simulink model "EVModeling"  (R2024b)
settings: Solver=ode23tb  StartTime=0  StopTime=1800  RelTol=1e-3
model workspace (MAT data in the model file):
  Af = Simulink.Parameter
  Af.Value = 2.27
  Af.Complexity = 'real'
  Af.Dimensions = [1 1]
  Af.DataType = 'double'
  Bx = Simulink.Parameter
  Bx.Value = 10
  Bx.Complexity = 'real'
  Bx.Dimensions = [1 1]
  Bx.DataType = 'double'
  CI = 0.1
  Cd = Simulink.Parameter
  Cd.Value = 0.28
  Cd.Complexity = 'real'
  Cd.Dimensions = [1 1]
  Cd.DataType = 'double'
  Cl = Simulink.Parameter
  Cl.Value = 0.1
  Cl.Complexity = 'real'
  Cl.Dimensions = [1 1]
  Cl.DataType = 'double'
  Cpm = Simulink.Parameter
  Cpm.Value = 0.1
  Cpm.Complexity = 'real'
  Cpm.Dimensions = [1 1]
  Cpm.DataType = 'double'
  Cx = Simulink.Parameter
  Cx.Value = 1.65
  Cx.Complexity = 'real'
  Cx.Dimensions = [1 1]
  Cx.DataType = 'double'
  Dx = Simulink.Parameter
  Dx.Value = 1
  Dx.Complexity = 'real'
  Dx.Dimensions = [1 1]
  Dx.DataType = 'double'
  Ex = Simulink.Parameter
  Ex.Value = 0.01
  Ex.Complexity = 'real'
  Ex.Dimensions = [1 1]
  Ex.DataType = 'double'
  FZMAX = Simulink.Parameter
  FZMAX.Value = 6570
  FZMAX.Complexity = 'real'
  FZMAX.Dimensions = [1 1]
  FZMAX.DataType = 'double'
  FZMIN = Simulink.Parameter
  FZMIN.Value = 0
  FZMIN.Complexity = 'real'
  FZMIN.Dimensions = [1 1]
  FZMIN.DataType = 'double'
  Fc = Simulink.Parameter
  Fc.Value = 500
  Fc.Complexity = 'real'
  Fc.Dimensions = [1 1]
  Fc.DataType = 'double'
  FsbF = Simulink.Parameter
  FsbF.Value = [-700000 -7000 -700 0 700 7000 700000]
  FsbF.Complexity = 'real'
  FsbF.Dimensions = [1 7]
  FsbF.DataType = 'double'
  FsbR = Simulink.Parameter
  FsbR.Value = [-700000 -7000 -700 0 700 7000 700000]
  FsbR.Complexity = 'real'
  FsbR.Dimensions = [1 7]
  FsbR.DataType = 'double'
  FskF = Simulink.Parameter
  FskF.Value = [-8928.57142857 -178.571428571 0 357.142857143 535.714285714 9285.71428571]
  FskF.Complexity = 'real'
  FskF.Dimensions = [1 6]
  FskF.DataType = 'double'
  FskR = Simulink.Parameter
  FskR.Value = [-5357.14285714 -107.142857143 0 214.285714286 321.428571429 5571.42857143]
  FskR.Complexity = 'real'
  FskR.Dimensions = [1 6]
  FskR.DataType = 'double'
  Iyy = Simulink.Parameter
  Iyy.Value = 3000
  Iyy.Complexity = 'real'
  Iyy.Dimensions = [1 1]
  Iyy.DataType = 'double'
  Iyy_Whl = Simulink.Parameter
  Iyy_Whl.Value = 0.8
  Iyy_Whl.Complexity = 'real'
  Iyy_Whl.Dimensions = [1 1]
  Iyy_Whl.DataType = 'double'
  J = Simulink.Parameter
  J.Value = 0.01
  J.Complexity = 'real'
  J.Dimensions = [1 1]
  J.DataType = 'double'
  Jd = Simulink.Parameter
  Jd.Value = 0.025
  Jd.Complexity = 'real'
  Jd.Dimensions = [1 1]
  Jd.DataType = 'double'
  Jmotor = Simulink.Parameter
  Jmotor.Value = 0.1
  Jmotor.Complexity = 'real'
  Jmotor.Dimensions = [1 1]
  Jmotor.DataType = 'double'
  Jw1 = Simulink.Parameter
  Jw1.Value = 0.01
  Jw1.Complexity = 'real'
  Jw1.Dimensions = [1 1]
  Jw1.DataType = 'double'
  Jw2 = Simulink.Parameter
  Jw2.Value = 0.01
  Jw2.Complexity = 'real'
  Jw2.Dimensions = [1 1]
  Jw2.DataType = 'double'
  Lrel = Simulink.Parameter
  Lrel.Value = 0.15
  Lrel.Complexity = 'real'
  Lrel.Dimensions = [1 1]
  Lrel.DataType = 'double'
  Mass = Simulink.Parameter
  Mass.Value = 1500
  Mass.Complexity = 'real'
  Mass.Dimensions = [1 1]
  Mass.DataType = 'double'
  NF = Simulink.Parameter
  NF.Value = 2
  NF.Complexity = 'real'
  NF.Dimensions = [1 1]
  NF.DataType = 'double'
  NR = Simulink.Parameter
  NR.Value = 2
  NR.Complexity = 'real'
  NR.Dimensions = [1 1]
  NR.DataType = 'double'
  Ndiff = Simulink.Parameter
  Ndiff.Value = 7.94
  Ndiff.Complexity = 'real'
  Ndiff.Dimensions = [1 1]
  Ndiff.DataType = 'double'
  Ndisks = Simulink.Parameter
  Ndisks.Value = 4
  Ndisks.Complexity = 'real'
  Ndisks.Dimensions = [1 1]
  Ndisks.DataType = 'double'
  Pabs = Simulink.Parameter
  Pabs.Value = 101325
  Pabs.Complexity = 'real'
  Pabs.Dimensions = [1 1]
  Pabs.DataType = 'double'
  Re = Simulink.Parameter
  Re.Value = 0.327
  Re.Complexity = 'real'
  Re.Dimensions = [1 1]
  Re.DataType = 'double'
  Reff_LSD = Simulink.Parameter
  Reff_LSD.Value = 0.2
  Reff_LSD.Complexity = 'real'
  Reff_LSD.Dimensions = [1 1]
  Reff_LSD.DataType = 'double'
  Rm = Simulink.Parameter
  Rm.Value = 0.15
  Rm.Complexity = 'real'
  Rm.Dimensions = [1 1]
  Rm.DataType = 'double'
  T = Simulink.Parameter
  T.Value = 273
  T.Complexity = 'real'
  T.Dimensions = [1 1]
  T.DataType = 'double'
  UNLOADED_RADIUS = Simulink.Parameter
  UNLOADED_RADIUS.Value = 0.336
  UNLOADED_RADIUS.Complexity = 'real'
  UNLOADED_RADIUS.Dimensions = [1 1]
  UNLOADED_RADIUS.DataType = 'double'
  VXLOW = Simulink.Parameter
  VXLOW.Value = 2
  VXLOW.Complexity = 'real'
  VXLOW.Dimensions = [1 1]
  VXLOW.DataType = 'double'
  aMy = Simulink.Parameter
  aMy.Value = 0.01
  aMy.Complexity = 'real'
  aMy.Dimensions = [1 1]
  aMy.DataType = 'double'
  a_CG = Simulink.Parameter
  a_CG.Value = 1.188
  a_CG.Complexity = 'real'
  a_CG.Dimensions = [1 1]
  a_CG.DataType = 'double'
  alphaMy = Simulink.Parameter
  alphaMy.Value = 0
  alphaMy.Complexity = 'real'
  alphaMy.Dimensions = [1 1]
  alphaMy.DataType = 'double'
  b = Simulink.Parameter
  b.Value = 400
  b.Complexity = 'real'
  b.Dimensions = [1 1]
  b.DataType = 'auto'
  b1 = Simulink.Parameter
  b1.Value = 100
  b1.Complexity = 'real'
  b1.Dimensions = [1 1]
  b1.DataType = 'double'
  bMy = Simulink.Parameter
  bMy.Value = 0
  bMy.Complexity = 'real'
  bMy.Dimensions = [1 1]
  bMy.DataType = 'double'
  b_CG = Simulink.Parameter
  b_CG.Value = 1.512
  b_CG.Complexity = 'real'
  b_CG.Dimensions = [1 1]
  b_CG.DataType = 'double'
  b_J = Simulink.Parameter
  b_J.Value = 0.001
  b_J.Complexity = 'real'
  b_J.Dimensions = [1 1]
  b_J.DataType = 'double'
  bd = Simulink.Parameter
  bd.Value = 0.001
  bd.Complexity = 'real'
  bd.Dimensions = [1 1]
  bd.DataType = 'double'
  betaMy = Simulink.Parameter
  betaMy.Value = 1
  betaMy.Complexity = 'real'
  betaMy.Dimensions = [1 1]
  betaMy.DataType = 'double'
  br = Simulink.Parameter
  br.Value = 0.001
  br.Complexity = 'real'
  br.Dimensions = [1 1]
  br.DataType = 'double'
  bw1 = Simulink.Parameter
  bw1.Value = 0.001
  bw1.Complexity = 'real'
  bw1.Dimensions = [1 1]
  bw1.DataType = 'double'
  bw2 = Simulink.Parameter
  bw2.Value = 0.001
  bw2.Complexity = 'real'
  bw2.Dimensions = [1 1]
  bw2.DataType = 'double'
  cMy = Simulink.Parameter
  cMy.Value = 0
  cMy.Complexity = 'real'
  cMy.Dimensions = [1 1]
  cMy.DataType = 'double'
  disk_abore = Simulink.Parameter
  disk_abore.Value = 0.05
  disk_abore.Complexity = 'real'
  disk_abore.Dimensions = [1 1]
  disk_abore.DataType = 'double'
  domega_o = Simulink.Parameter
  domega_o.Value = 0
  domega_o.Complexity = 'real'
  domega_o.Dimensions = [1 1]
  domega_o.DataType = 'double'
  dw = Simulink.Parameter
  dw.Value = [0 10 20 40 60 80 100]
  dw.Complexity = 'real'
  dw.Dimensions = [1 7]
  dw.DataType = 'double'
  dzdotsF = Simulink.Parameter
  dzdotsF.Value = [-10 -1 -0.1 0 0.1 1 10]
  dzdotsF.Complexity = 'real'
  dzdotsF.Dimensions = [1 7]
  dzdotsF.DataType = 'double'
  dzdotsR = Simulink.Parameter
  dzdotsR.Value = [-10 -1 -0.1 0 0.1 1 10]
  dzdotsR.Complexity = 'real'
  dzdotsR.Dimensions = [1 7]
  dzdotsR.DataType = 'double'
  dzsF = Simulink.Parameter
  dzsF.Value = [-0.005 -0.0001 0 0.2 0.2001 0.2051]
  dzsF.Complexity = 'real'
  dzsF.Dimensions = [1 6]
  dzsF.DataType = 'double'
  dzsR = Simulink.Parameter
  dzsR.Value = [-0.005 -0.0001 0 0.2 0.2001 0.2051]
  dzsR.Complexity = 'real'
  dzsR.Dimensions = [1 6]
  dzsR.DataType = 'double'
  g = Simulink.Parameter
  g.Value = 9.81
  g.Complexity = 'real'
  g.Dimensions = [1 1]
  g.DataType = 'double'
  h = Simulink.Parameter
  h.Value = 0.5
  h.Complexity = 'real'
  h.Dimensions = [1 1]
  h.DataType = 'double'
  k = Simulink.Parameter
  k.Value = 10000
  k.Complexity = 'real'
  k.Dimensions = [1 1]
  k.DataType = 'auto'
  k1 = Simulink.Parameter
  k1.Value = 50000
  k1.Complexity = 'real'
  k1.Dimensions = [1 1]
  k1.DataType = 'double'
  kappamax = Simulink.Parameter
  kappamax.Value = 1.5
  kappamax.Complexity = 'real'
  kappamax.Dimensions = [1 1]
  kappamax.DataType = 'double'
  lam_x = Simulink.Parameter
  lam_x.Value = 1
  lam_x.Complexity = 'real'
  lam_x.Dimensions = [1 1]
  lam_x.DataType = 'double'
  mu_kinetic = Simulink.Parameter
  mu_kinetic.Value = 0.35
  mu_kinetic.Complexity = 'real'
  mu_kinetic.Dimensions = [1 1]
  mu_kinetic.DataType = 'double'
  mu_static = Simulink.Parameter
  mu_static.Value = 0.45
  mu_static.Complexity = 'real'
  mu_static.Dimensions = [1 1]
  mu_static.DataType = 'double'
  muc = Simulink.Parameter
  muc.Value = [0.16 0.13 0.115 0.11 0.105 0.1025 0.10125]
  muc.Complexity = 'real'
  muc.Dimensions = [1 7]
  muc.DataType = 'double'
  num_pads = Simulink.Parameter
  num_pads.Value = 2
  num_pads.Complexity = 'real'
  num_pads.Dimensions = [1 1]
  num_pads.DataType = 'double'
  omega1_c = Simulink.Parameter
  omega1_c.Value = 3000
  omega1_c.Complexity = 'real'
  omega1_c.Dimensions = [1 1]
  omega1_c.DataType = 'double'
  omega_c = Simulink.Parameter
  omega_c.Value = 100
  omega_c.Complexity = 'real'
  omega_c.Dimensions = [1 1]
  omega_c.DataType = 'auto'
  omega_o = Simulink.Parameter
  omega_o.Value = 0
  omega_o.Complexity = 'real'
  omega_o.Dimensions = [1 1]
  omega_o.DataType = 'double'
  omega_o_J = Simulink.Parameter
  omega_o_J.Value = 0
  omega_o_J.Complexity = 'real'
  omega_o_J.Dimensions = [1 1]
  omega_o_J.DataType = 'double'
  omegao = Simulink.Parameter
  omegao.Value = 0
  omegao.Complexity = 'real'
  omegao.Dimensions = [1 1]
  omegao.DataType = 'double'
  omegaw1o = Simulink.Parameter
  omegaw1o.Value = 0
  omegaw1o.Complexity = 'real'
  omegaw1o.Dimensions = [1 1]
  omegaw1o.DataType = 'double'
  omegaw2o = Simulink.Parameter
  omegaw2o.Value = 0
  omegaw2o.Complexity = 'real'
  omegaw2o.Dimensions = [1 1]
  omegaw2o.DataType = 'double'
  press = Simulink.Parameter
  press.Value = 234400
  press.Complexity = 'real'
  press.Dimensions = [1 1]
  press.DataType = 'double'
  q_o = Simulink.Parameter
  q_o.Value = 0
  q_o.Complexity = 'real'
  q_o.Dimensions = [1 1]
  q_o.DataType = 'double'
  tauC_LSD = Simulink.Parameter
  tauC_LSD.Value = 0.01
  tauC_LSD.Complexity = 'real'
  tauC_LSD.Dimensions = [1 1]
  tauC_LSD.DataType = 'double'
  theta_o = Simulink.Parameter
  theta_o.Value = 0
  theta_o.Complexity = 'real'
  theta_o.Dimensions = [1 1]
  theta_o.DataType = 'double'
  theta_o_Veh = Simulink.Parameter
  theta_o_Veh.Value = 0
  theta_o_Veh.Complexity = 'real'
  theta_o_Veh.Dimensions = [1 1]
  theta_o_Veh.DataType = 'double'
  wc_shaft = Simulink.Parameter
  wc_shaft.Value = 0.1
  wc_shaft.Complexity = 'real'
  wc_shaft.Dimensions = [1 1]
  wc_shaft.DataType = 'auto'
  x_o = Simulink.Parameter
  x_o.Value = 0
  x_o.Complexity = 'real'
  x_o.Dimensions = [1 1]
  x_o.DataType = 'double'
  xdot_o = Simulink.Parameter
  xdot_o.Value = 0
  xdot_o.Complexity = 'real'
  xdot_o.Dimensions = [1 1]
  xdot_o.DataType = 'double'
  z_o = Simulink.Parameter
  z_o.Value = -0.35
  z_o.Complexity = 'real'
  z_o.Dimensions = [1 1]
  z_o.DataType = 'double'
  zdot_o = Simulink.Parameter
  zdot_o.Value = 0
  zdot_o.Complexity = 'real'
  zdot_o.Dimensions = [1 1]
  zdot_o.DataType = 'double'
undefined symbols (not defined in the file): DiscIntNeverNeededParam
libraries: autolibshared x5, autolibsharedcoupling x3, autolibpowerinfoutils x2, autolibshareddiff x1
(part 1 of 3)
settings Model: SimulationMode=accelerator  Creator=jungj  LastModifiedBy=jungj
settings SolverCC: ZeroCrossAlgorithm=Adaptive  AutoInsertRateTranBlk=on
settings ModelReferenceCC: UpdateModelReferenceTargets=IfOutOfDate  EnableRefExpFcnMdlSchedulingChecks=on  ModelReferenceMinAlgLoopOccurrences=on  PropagateSignalLabelsOutOfModel=off

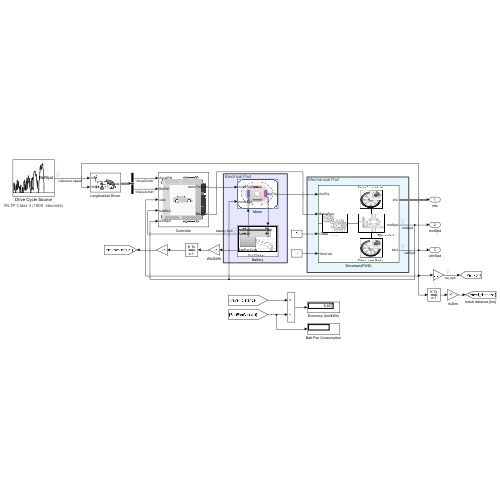
[thumbnail: Simulink's stored preview of the top-level diagram]
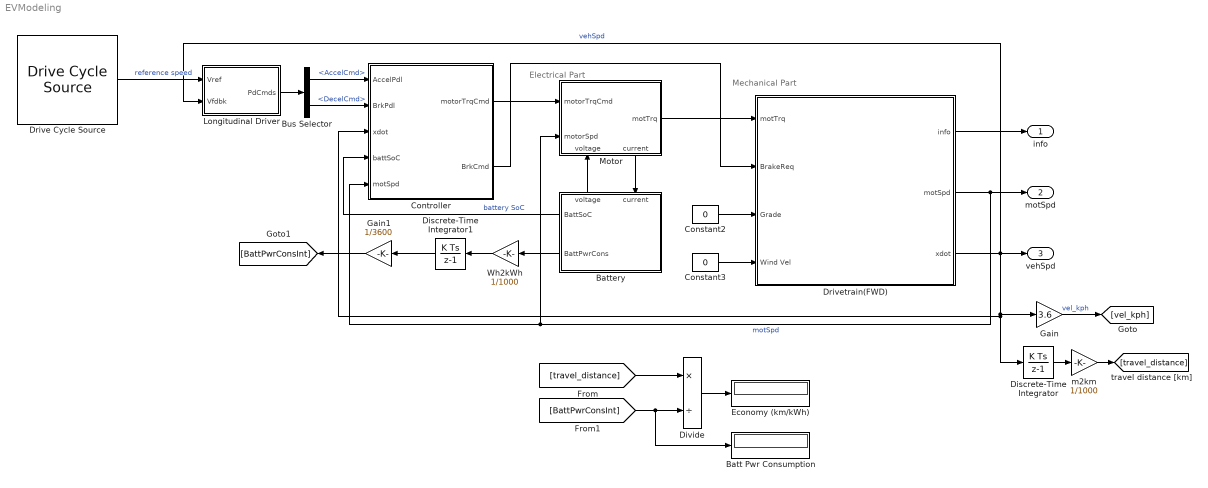
== system EVModeling ==
  note: Mechanical Part
  note: Electrical Part
  Batt Pwr Consumption : Display
  Battery : Subsystem
      settings: PortSchema="{\"entries\":[{\"content\":{\"sides\":[{\"content\":{\"connectorIds\":[\"Out2\",\"Out3\"]},\"type\":\"ConnectorPlacement.EquallySpacedRectSide\",\"uuid\":\"c2bfbeae-3225-4f42-88d6-04d8f56de19d\"},{\"content\":{\"side\":\"RIGHT\"},\"type\":\"ConnectorPlacement.EquallySpacedRectSide\",\"uuid\":\"8167ae6e-a28c-428b-8858-a507e5bff4d9\"},{\"content\":{\"connectorIds\":[\"Out1\",\"In1\"],\"side\":\"TOP\"},\"type\":\"ConnectorPlacement.EquallySpacedRectSide\",\"uuid\":\"2ce101ba-922d-478b-940c-623fe876fa36\"}]},\"type\":\"ConnectorPlacement.EquallySpacedConnector\",\"uuid\":\"864f1a3d-41ce-48bc-9e39-bda578cb0e6c\"}],\"packageUris\":[\"http://schema.mathworks.com/mf0/Connector/R2020b\"],\"version\":\"1.0\"}"
      mask Display: image('battery.png');
  Bus Selector : BusSelector  OutputSignals=AccelCmd,DecelCmd
  Constant2 : Constant  Value=0
  Constant3 : Constant  Value=0
  Controller : Subsystem
      mask Display: image('SystemControllers.png');
  Discrete-Time Integrator : DiscreteIntegrator  SampleTime=-1  ICPrevOutput=DiscIntNeverNeededParam  ICPrevScaledInput=DiscIntNeverNeededParam
  Discrete-Time Integrator1 : DiscreteIntegrator  SampleTime=-1  ICPrevOutput=DiscIntNeverNeededParam  ICPrevScaledInput=DiscIntNeverNeededParam
  Divide : Product  Inputs=*/
  Drive Cycle Source : autolibshared/Drive Cycle Source  cycleVar=WLTP Class 3  fileVar=cycleFTP75.mat  tfinal="1800  seconds"  cycleRepeat=off  outAccPort=off  outGearPort=off  gearList=No gear data  t_wot1=5  xdot_woto=0  xdot_wot1=30  t_wot2=20  xdot_wot2=0  t_wotend=30  srcUnit=m/s  outUnit=m/s  srcAccUnit=m/s/s  outAccUnit=m/s^2  dt=0  aMode=1  faultOption=off  velBnd=2  velBndUnit=mph  inUnit=m/s  timeBnd=1  failOption=off  stopSim=off  maxFaultCnt=10  maxFaultTime=2  maxTotFaultTime=15  traceOption=off  dtTrace=1  traceWindow=10  lastDCname=WLTP Class 3  lastOutUnit=mph  lastDT=0  lastTB=1  lastSB=2  forceCalcBound=off
  Drivetrain(FWD) : Subsystem
      mask Display: image('mechanicalPart.png');
  Economy (km/kWh) : Display
  Gain : Gain  Gain=3.6
  Gain1 : Gain  Gain=1/3600
  Longitudinal Driver : Subsystem
      mask Display: image('LongitudinalDriver.png');
  Motor : Subsystem
      settings: PortSchema="{\"entries\":[{\"content\":{\"sides\":[{\"content\":{\"connectorIds\":[\"In1\",\"In2\"]},\"type\":\"ConnectorPlacement.EquallySpacedRectSide\",\"uuid\":\"07a928c4-0315-47a5-8fbb-db51356538de\"},{\"content\":{\"connectorIds\":[\"Out1\"],\"side\":\"RIGHT\"},\"type\":\"ConnectorPlacement.EquallySpacedRectSide\",\"uuid\":\"1e6f9828-2a39-4883-95b5-e401da73848e\"},{\"content\":{\"side\":\"TOP\"},\"type\":\"ConnectorPlacement.EquallySpacedRectSide\",\"uuid\":\"3ae8d425-af29-4da6-9a06-f6979c9afd20\"},{\"content\":{\"connectorIds\":[\"In3\",\"Out2\"],\"side\":\"BOTTOM\"},\"type\":\"ConnectorPlacement.EquallySpacedRectSide\",\"uuid\":\"6bdfdf60-af65-44a3-8b94-a2f6402ffb18\"}]},\"type\":\"ConnectorPlacement.EquallySpacedConnector\",\"uuid\":\"e18243ef-e83a-4e85-b843-3cc44aad2b17\"}],\"packageUris\":[\"http://schema.mathworks.com/mf0/Connector/R2020b\"],\"version\":\"1.0\"}"
      mask Display: image('motor.png');
  Wh2kWh : Gain  Gain=1/1000
  m2km : Gain  Gain=1/1000
  info : Outport
  motSpd : Outport  Port=2
  vehSpd : Outport  Port=3
  wires:
  Constant2/1 -> Drivetrain(FWD)/3(Grade)
  Constant3/1 -> Drivetrain(FWD)/4(Wind Vel)
  Drivetrain(FWD)/1(info) -> info/1
  Drivetrain(FWD)/2(motSpd) -> Motor/2(motorSpd), Controller/5(motSpd), motSpd/1  "motSpd"
  Drivetrain(FWD)/3(xdot) -> Discrete-Time Integrator/1, Controller/3(xdot), Gain/1, Longitudinal Driver/2(Vfdbk), vehSpd/1  "vehSpd"
  Motor/1(motTrq) -> Drivetrain(FWD)/1(motTrq)
  Controller/1(motorTrqCmd) -> Motor/1(motorTrqCmd)
  Controller/2(BrkCmd) -> Drivetrain(FWD)/2(BrakeReq)
  Drive Cycle Source/1 -> Longitudinal Driver/1(Vref)  "reference speed"
  Battery/1(voltage) -> Motor/3(voltage)
  Motor/2(current) -> Battery/1(current)
  Longitudinal Driver/1(PdCmds) -> Bus Selector/1
  Bus Selector/1 -> Controller/1(AccelPdl)  "<AccelCmd>"
  Bus Selector/2 -> Controller/2(BrkPdl)  "<DecelCmd>"
  Battery/2(BattSoC) -> Controller/4(battSoC)  "battery SoC"
  Gain/1 -> [vel_kph]  "vel_kph"
  [travel_distance] -> Divide/1
  [BattPwrConsInt] -> Batt Pwr Consumption/1, Divide/2
  Divide/1 -> Economy (km/kWh)/1
  Discrete-Time Integrator/1 -> m2km/1
  m2km/1 -> [travel_distance]
  Battery/3(BattPwrCons) -> Wh2kWh/1
  Wh2kWh/1 -> Discrete-Time Integrator1/1
  Discrete-Time Integrator1/1 -> Gain1/1
  Gain1/1 -> [BattPwrConsInt]

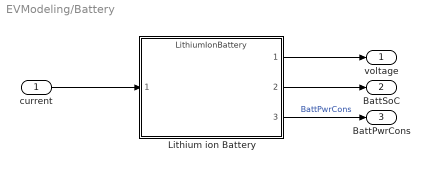
== system EVModeling/Battery ==
  current : Inport
  Lithium ion Battery : ModelReference  ModelNameDialog=LithiumIonBattery.slx  SimulationMode=Normal  ModelReferenceVersion=1.8
  voltage : Outport
  BattSoC : Outport  Port=2
  BattPwrCons : Outport  Port=3
  wires:
  Lithium ion Battery/2 -> BattSoC/1
  Lithium ion Battery/1 -> voltage/1
  current/1 -> Lithium ion Battery/1
  Lithium ion Battery/3 -> BattPwrCons/1  "BattPwrCons"

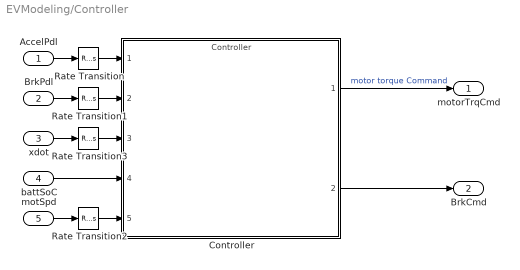
== system EVModeling/Controller ==
  AccelPdl : Inport
  BrkPdl : Inport  Port=2
  xdot : Inport  Port=3
  battSoC : Inport  Port=4
  motSpd : Inport  Port=5
  Controller : ModelReference  ModelNameDialog=Controller.slx  SimulationMode=Normal  ModelReferenceVersion=1.79
  Rate Transition{,1..3} (4 alike) : RateTransition  Deterministic=off
  motorTrqCmd : Outport
  BrkCmd : Outport  Port=2
  wires:
  Controller/1 -> motorTrqCmd/1  "motor torque Command"
  Controller/2 -> BrkCmd/1
  AccelPdl/1 -> Rate Transition/1
  BrkPdl/1 -> Rate Transition1/1
  xdot/1 -> Rate Transition3/1
  battSoC/1 -> Controller/4
  motSpd/1 -> Rate Transition2/1
  Rate Transition/1 -> Controller/1
  Rate Transition1/1 -> Controller/2
  Rate Transition2/1 -> Controller/5
  Rate Transition3/1 -> Controller/3

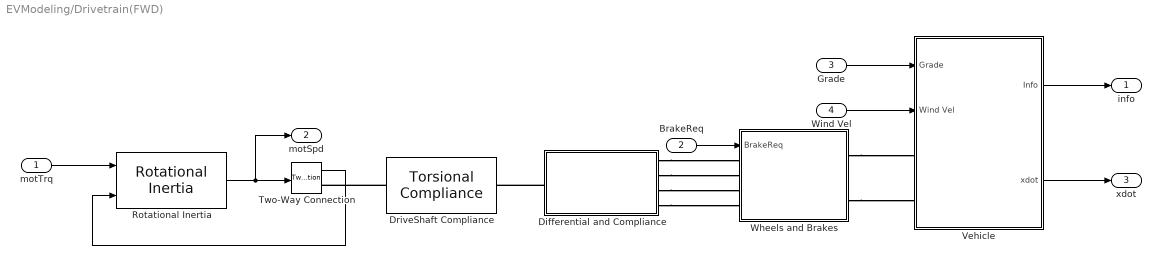
== system EVModeling/Drivetrain(FWD) ==
  motTrq : Inport
  BrakeReq : Inport  Port=2
  Grade : Inport  Port=3
  Wind Vel : Inport  Port=4
  Differential and Compliance : Subsystem
  DriveShaft Compliance : autolibsharedcoupling/Torsional Compliance  port_config=Two-way connection  extInfo=off  k=k  b=b  theta_o=theta_o  domega_o=domega_o  omega_c=omega_c  blkID=0  aMode=1
  Rotational Inertia : autolibsharedcoupling/Rotational Inertia  port_config=Simulink  extInfo=off  externJ=off  J=Jmotor  b=.001  omega_o=omega_o  blkID=0  aMode=1
      settings: LibrarySourceBlock=autolibcoupling/Rotational Inertia
  Two-Way Connection : TwoWayConnection
  Vehicle : Subsystem
  Wheels and Brakes : Subsystem  VariantControl=0
  info : Outport
  motSpd : Outport  Port=2
  xdot : Outport  Port=3
  wires:
  motTrq/1 -> Rotational Inertia/1
  Rotational Inertia/1 -> motSpd/1, Two-Way Connection/1
  Two-Way Connection/1 -> Rotational Inertia/2
  Wind Vel/1 -> Vehicle/2(Wind Vel)
  Grade/1 -> Vehicle/1(Grade)
  BrakeReq/1 -> Wheels and Brakes/1(BrakeReq)
  Vehicle/1(Info) -> info/1
  Vehicle/2(xdot) -> xdot/1
  connections:
  DriveShaft Compliance/LConn1 -- Two-Way Connection/RConn1
  Differential and Compliance/LConn1 -- DriveShaft Compliance/RConn1
  Differential and Compliance/RConn1 -- Wheels and Brakes/LConn1
  Differential and Compliance/RConn2 -- Wheels and Brakes/LConn2
  Differential and Compliance/RConn3 -- Wheels and Brakes/LConn3
  Differential and Compliance/RConn4 -- Wheels and Brakes/LConn4
  Wheels and Brakes/RConn1 -- Vehicle/LConn1
  Wheels and Brakes/RConn2 -- Vehicle/LConn2

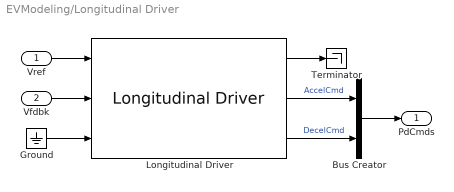
== system EVModeling/Longitudinal Driver ==
  Vref : Inport
  Vfdbk : Inport  Port=2
  Bus Creator : BusCreator  Inputs=2
  Ground : Ground
  Longitudinal Driver : autolibshared/Longitudinal Driver  extAccelOvr=off  extDecelOvr=off  extAccelHld=off  extDecelHld=off  extAccelZero=off  extDecelZero=off  cntrlType=Predictive  shftType=Reverse, Neutral, Drive  velUnits=m/s  gearOut=off  Kp=15  Ki=1  Kff=.05  Kg=.01  VehVelVec=[0 100]  KffVec=[.1 .1]  KpVec=[10 10]  KiVec=[5 5]  KgVec=[0 0]  m=1645  Kpt=450*9.04/0.324  tau=.12  L=4  aR=30.3/3875  bR=0.21290*4.44822/0.44704  cR=0.01278*4.44822/0.44704^2  g=9.81  vnom=100  Kaw=.1  tauerr=.03  tauPt=2  GearInit=0  tShift=.1  pdlVec=[0.1 0.4 0.5 0.9]  upShftTbl=[-1 12.9375 26.4375 39.9375 51.18749999999999 62.4375 72.84375 83.25;-1 16.3125 29.8125 43.3125 54.5624 65.8125 76.78125 87.75;-1 19.6875 33.1875 46.68749999999999 57.9375 69.1875 80.71875 92.25;-1 33 52.5 77.25 100.5 138.75 161.875 185]  dwnShftTbl=[1 9.5625 23.0625 36.5625 47.8125 59.0625 68.90625 78.75;1 12.9375 26.4375 39.9375 51.18749999999999 62.4375 72.84375 83.25;1 16.3125 29.8125 43.3125 54.562499 65.8125 76.78125 87.75;1 19.6875 33.1875 46.68749999999999 57.9375 69.1875 80.71875 92.25]  tClutch=.5  tRev=.5  tPark=120  aMode=1  UpGearVec="[0  1  2  3  4  5  6  7]"  DownGearVec="[1  2  3  4  5  6  7  8]"
  Terminator : Terminator
  PdCmds : Outport
  wires:
  Vref/1 -> Longitudinal Driver/1
  Vfdbk/1 -> Longitudinal Driver/2
  Ground/1 -> Longitudinal Driver/3
  Longitudinal Driver/2 -> Bus Creator/1  "AccelCmd"
  Longitudinal Driver/3 -> Bus Creator/2  "DecelCmd"
  Bus Creator/1 -> PdCmds/1
  Longitudinal Driver/1 -> Terminator/1

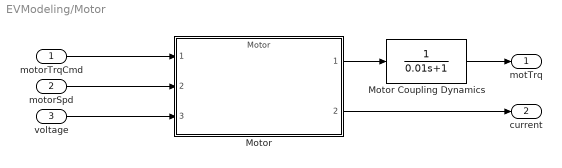
== system EVModeling/Motor ==
  motorTrqCmd : Inport
  motorSpd : Inport  Port=2
  voltage : Inport  Port=3
  Motor : ModelReference  ModelNameDialog=Motor.slx  SimulationMode=Normal  ModelReferenceVersion=1.5
  Motor Coupling Dynamics : TransferFcn  Denominator=[0.01 1]
  motTrq : Outport
  current : Outport  Port=2
  wires:
  motorSpd/1 -> Motor/2
  voltage/1 -> Motor/3
  motorTrqCmd/1 -> Motor/1
  Motor/1 -> Motor Coupling Dynamics/1
  Motor/2 -> current/1
  Motor Coupling Dynamics/1 -> motTrq/1

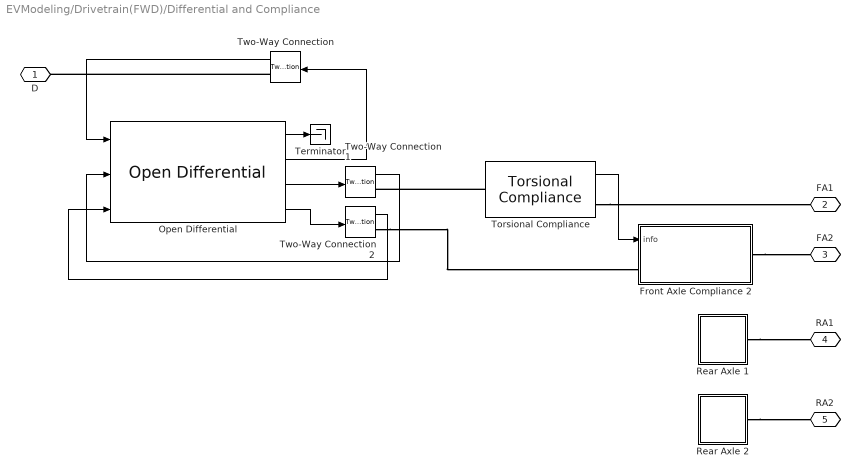
== system EVModeling/Drivetrain(FWD)/Differential and Compliance ==
  Front Axle Compliance 2 : Subsystem
  Open Differential : autolibshareddiff/Open Differential  DiffEffModelPopup=Constant  InterpMethod=Linear point-slope  extTamb=off  shaftSwitchMask=To the left of center-line  Ndiff=Ndiff  Jd=Jd  bd=bd  Jw1=Jw1  bw1=bw1  Jw2=Jw2  bw2=bw2  omegaw1o=omegaw1o  omegaw2o=omegaw2o  eta=1  eta_tbl=reshape([0.64 0.76 0.8 0.81 0.83 0.84 0.84 0.56 0.73 0.78 0.8 0.83 0.84 0.84 0.54 0.71 0.77 0.8 0.82 0.84 0.84 0.53 0.71 0.77 0.8 0.83 0.84 0.84 0.51 0.71 0.77 0.8 0.83 0.84 0.85 0.52 0.7 0.77 0.8 0.83 0.84 0.85 0.51 0.71 0.76 0.79 0.83 0.84 0.85 0.5 0.69 0.76 0.79 0.82 0.84 0.85 0.45 0.68 0.75 0.78 0.82 0.84 0.85 0.43 0.67 0.74 0.78 0.81 0.83 0.84 0.38 0.63 0.71 0.75 0.8 0.82 0.83 0.81 0.86 0.88 0.89 0.89 0.89 0.9 0.77 0.85 0.87 0.88 0.89 0.9 0.9 0.72 0.82 0.86 0.87 0.88 0.89 0.9 0.68 0.8 0.84 0.86 0.88 0.89 0.89 0.67 0.8 0.84 0.86 0.88 0.89 0.9 0.67 0.8 0.84 0.86 0.88 0.89 0.9 0.65 0.8 0.84 0.86 0.88 0.89 0.9 0.64 0.79 0.83 0.86 0.88 0.89 0.9 0.63 0.78 0.83 0.86 0.88 0.89 0.9 0.59 0.76 0.82 0.85 0.87 0.89 0.9 0.53 0.73 0.8 0.83 0.86 0.88 0.89], 7, 11, 2)  Trq_bpts=[25, 50, 75, 100, 150, 200, 250]  omega_bpts=[52.4 78.5 105 131 157 183 209 262 314 419 524]  Temp_bpts=[290 358]  Tamb=297.15  maxAbsSpd=5e3  aMode=1
      settings: LibrarySourceBlock=autolibdiff/Open Differential
  Rear Axle 1 : Subsystem
  Rear Axle 2 : Subsystem
  Terminator : Terminator
  Torsional Compliance : autolibsharedcoupling/Torsional Compliance  port_config=Two-way connection  extInfo=on  k=k  b=b  theta_o=theta_o  domega_o=domega_o  omega_c=omega_c  blkID=0  aMode=1
  Two-Way Connection : TwoWayConnection
  Two-Way Connection1 : TwoWayConnection
  Two-Way Connection2 : TwoWayConnection
  D : PMIOPort  Side=Left
  FA1 : PMIOPort  Port=2  Side=Right
  FA2 : PMIOPort  Port=3  Side=Right
  RA1 : PMIOPort  Port=4  Side=Right
  RA2 : PMIOPort  Port=5  Side=Right
  wires:
  Two-Way Connection/1 -> Open Differential/1
  Open Differential/2 -> Two-Way Connection/1
  Open Differential/3 -> Two-Way Connection1/1
  Open Differential/4 -> Two-Way Connection2/1
  Two-Way Connection1/1 -> Open Differential/2
  Two-Way Connection2/1 -> Open Differential/3
  Open Differential/1 -> Terminator/1
  Torsional Compliance/1 -> Front Axle Compliance 2/1(info)
  connections:
  Two-Way Connection/RConn1 -- D/RConn1
  Torsional Compliance/LConn1 -- Two-Way Connection1/RConn1
  Torsional Compliance/RConn1 -- FA1/RConn1
  Front Axle Compliance 2/RConn1 -- FA2/RConn1
  Two-Way Connection2/RConn1 -- Front Axle Compliance 2/LConn1
  Rear Axle 1/RConn1 -- RA1/RConn1
  Rear Axle 2/RConn1 -- RA2/RConn1

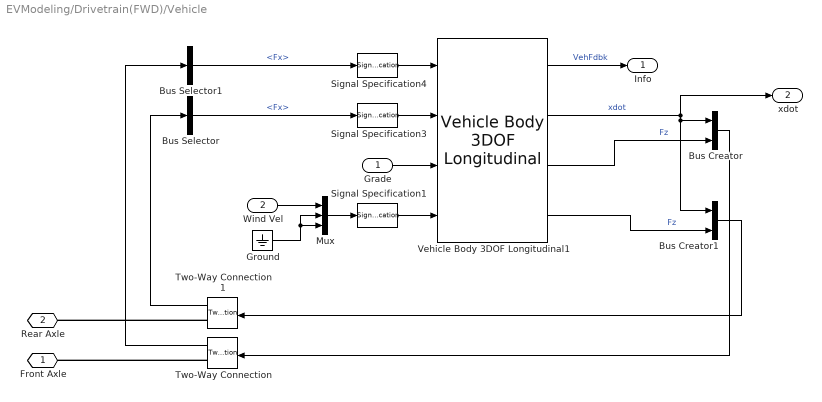
== system EVModeling/Drivetrain(FWD)/Vehicle ==
  Grade : Inport  Unit=deg
  Wind Vel : Inport  Port=2  Unit=m/s
  Bus Creator : BusCreator  Inputs=2
  Bus Creator1 : BusCreator  Inputs=2
  Bus Selector : BusSelector  OutputSignals=Fx
  Bus Selector1 : BusSelector  OutputSignals=Fx
  Ground : Ground
  Mux : Mux  Inputs=3
  Signal Specification1 : SignalSpecification  Unit=m/s
  Signal Specification3 : SignalSpecification  Unit=N
  Signal Specification4 : SignalSpecification  Unit=N
  Two-Way Connection : TwoWayConnection
  Two-Way Connection1 : TwoWayConnection
  Vehicle Body 3DOF Longitudinal1 : autolibshared/Vehicle Body 3DOF Longitudinal  VariantControl=SL  groundType=Grade angle  aMode=1  extFMode=off  extMMode=off  extTamb=off  NF=NF  NR=NR  m=Mass  a=a_CG  b=b_CG  h=h  Cd=Cd  Af=Af  x_o=x_o  xdot_o=xdot_o  Cl=CI  z_o=z_o  zdot_o=zdot_o  Iyy=Iyy  Cpm=Cpm  theta_o=theta_o_Veh  q_o=q_o  FskF=FskF  dzsF=dzsF  FsbF=FsbF  dzdotsF=dzdotsF  FskR=FskR  dzsR=dzsR  FsbR=FsbR  dzdotsR=dzdotsR  Pabs=Pabs  T=T  g=g  blkID=0
      settings: LibrarySourceBlock=autolibvehdynlong/Vehicle Body 3DOF Longitudinal
  Front Axle : PMIOPort  Side=Left
  Rear Axle : PMIOPort  Port=2  Side=Left
  Info : Outport  VectorParamsAs1DForOutWhenUnconnected=off
  xdot : Outport  Port=2
  wires:
  Signal Specification3/1 -> Vehicle Body 3DOF Longitudinal1/2
  Vehicle Body 3DOF Longitudinal1/2 -> Bus Creator1/1, Bus Creator/1, xdot/1  "xdot"
  Vehicle Body 3DOF Longitudinal1/3 -> Bus Creator/2  "Fz"
  Vehicle Body 3DOF Longitudinal1/4 -> Bus Creator1/2  "Fz"
  Bus Creator1/1 -> Two-Way Connection1/1
  Bus Creator/1 -> Two-Way Connection/1
  Two-Way Connection1/1 -> Bus Selector/1
  Bus Selector/1 -> Signal Specification3/1  "<Fx>"
  Bus Selector1/1 -> Signal Specification4/1  "<Fx>"
  Two-Way Connection/1 -> Bus Selector1/1
  Wind Vel/1 -> Mux/1
  Ground/1 -> Mux/3, Mux/2
  Mux/1 -> Signal Specification1/1
  Vehicle Body 3DOF Longitudinal1/1 -> Info/1  "VehFdbk"
  Grade/1 -> Vehicle Body 3DOF Longitudinal1/3
  Signal Specification1/1 -> Vehicle Body 3DOF Longitudinal1/4
  Signal Specification4/1 -> Vehicle Body 3DOF Longitudinal1/1
  connections:
  Two-Way Connection/RConn1 -- Front Axle/RConn1
  Two-Way Connection1/RConn1 -- Rear Axle/RConn1
